simulink model "Scenario_MinimumExample_TwithoutTrafficLights_tol_fixed"  (R2021a)
settings: Solver=VariableStepAuto  StartTime=0.0  StopTime=50  RelTol=1e-3
model workspace (MAT data in the model file):
  Kz_dif : Simulink.Parameter (value not decoded)
  Kz_il : Simulink.Parameter (value not decoded)
  Kz_ir : Simulink.Parameter (value not decoded)
  Kz_is : Simulink.Parameter (value not decoded)
  Kz_long : Simulink.Parameter (value not decoded)
  Kz_pre : Simulink.Parameter (value not decoded)
  L_dif : Simulink.Parameter (value not decoded)
  L_il : Simulink.Parameter (value not decoded)
  L_ir : Simulink.Parameter (value not decoded)
  L_is : Simulink.Parameter (value not decoded)
  L_long : Simulink.Parameter (value not decoded)
  L_pre : Simulink.Parameter (value not decoded)
  Lc : Simulink.Parameter (value not decoded)
  Rk : Simulink.Parameter (value not decoded)
  Tz_dif : Simulink.Parameter (value not decoded)
  Tz_il : Simulink.Parameter (value not decoded)
  Tz_ir : Simulink.Parameter (value not decoded)
  Tz_is : Simulink.Parameter (value not decoded)
  Tz_long : Simulink.Parameter (value not decoded)
  Tz_pre : Simulink.Parameter (value not decoded)
  ds : Simulink.Parameter (value not decoded)
  dt : Simulink.Parameter (value not decoded)
  v : Simulink.Parameter (value not decoded)
symbols that are objects in the model workspace (value not decoded): Kz_dif, Kz_il, Kz_ir, Kz_is, Kz_long, Kz_pre, Rk, Tz_dif, Tz_il, Tz_ir, Tz_is, Tz_long, Tz_pre
libraries: StreetLanesLibrary x72, EdgesLibrary x64, MeasuringLibrary x34, SourcesAndSinksLibrary x11
(part 2 of 3)

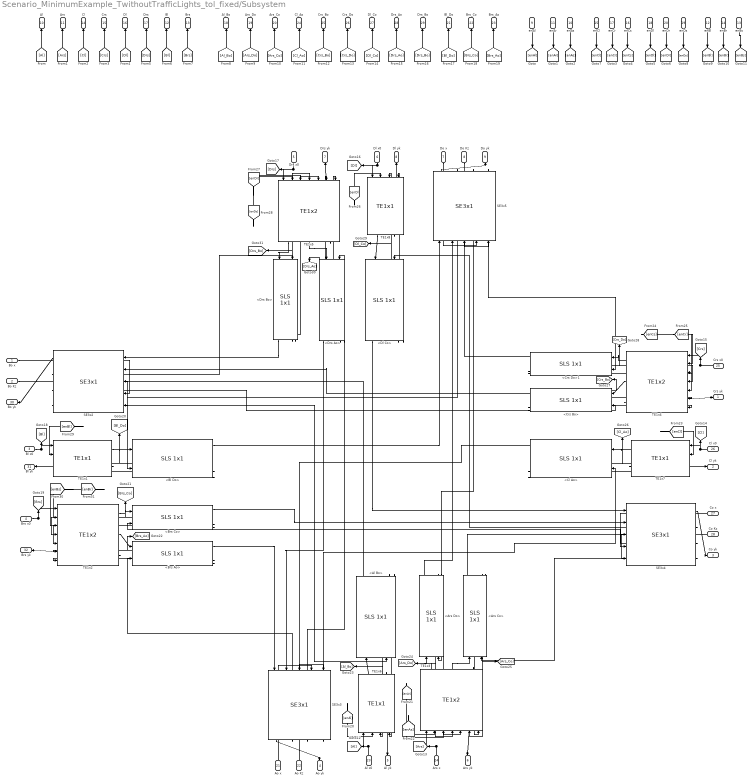
== system Scenario_MinimumExample_TwithoutTrafficLights_tol_fixed/Subsystem ==
  Bo x : Inport
  Bo Kz : Inport  Port=2
  Bl x0 : Inport  Port=3
  Brs x0 : Inport  Port=4
  Drs x0 : Inport  Port=5
  Dl x0 : Inport  Port=6
  Do x : Inport  Port=7
  Do Kz : Inport  Port=8
  enAl : Inport  Port=9
  enAs : Inport  Port=10
  enAr : Inport  Port=11
  enBl : Inport  Port=12
  enBs : Inport  Port=13
  enBr : Inport  Port=14
  enCl : Inport  Port=15
  enCs : Inport  Port=16
  enCr : Inport  Port=17
  enDl : Inport  Port=18
  enDs : Inport  Port=19
  enDr : Inport  Port=20
  Ao x : Inport  Port=21
  Ao Kz : Inport  Port=22
  Al x0 : Inport  Port=23
  Ars x : Inport  Port=24
  Crs x0 : Inport  Port=25
  Cl x0 : Inport  Port=26
  Co x : Inport  Port=27
  Co Kz : Inport  Port=28
  <Al Bo> : StreetLanesLibrary/SLS 1x1  Kz=Kz_left  Tz=Tz_left
  <Ars Co> : StreetLanesLibrary/SLS 1x1  Kz=Kz_right  Tz=Tz_right
  <Ars Do> : StreetLanesLibrary/SLS 1x1  Kz=Kz_straight  Tz=Tz_straight
  <Bl Do> : StreetLanesLibrary/SLS 1x1  Kz=Kz_left  Tz=Tz_left
  <Brs Ao> : StreetLanesLibrary/SLS 1x1  Kz=Kz_right  Tz=Tz_right
  <Brs Co> : StreetLanesLibrary/SLS 1x1  Kz=Kz_straight  Tz=Tz_straight
  <Cl Ao> : StreetLanesLibrary/SLS 1x1  Kz=Kz_left  Tz=Tz_left
  <Crs Bo> : StreetLanesLibrary/SLS 1x1  Kz=Kz_straight  Tz=Tz_straight
  <Crs Do>1 : StreetLanesLibrary/SLS 1x1  Kz=Kz_right  Tz=Tz_right
  <Dl Co> : StreetLanesLibrary/SLS 1x1  Kz=Kz_left  Tz=Tz_left
  <Drs Ao> : StreetLanesLibrary/SLS 1x1  Kz=Kz_straight  Tz=Tz_straight
  <Drs Bo> : StreetLanesLibrary/SLS 1x1  Kz=Kz_right  Tz=Tz_right
  SE3x{2..5} (4 alike) : EdgesLibrary/SE3x1  Rk1=Rk  Rk2=Rk  Rk3=Rk
  TE1x{1,6..8} (4 alike) : EdgesLibrary/TE1x1  Rk=Rk  slope=2000
  TE1x{2..5} (4 alike) : EdgesLibrary/TE1x2  Rk1=0.5*Rk  Rk2=0.5*Rk
  Crs yk : Outport
  Cl yk : Outport  Port=2
  Co yk : Outport  Port=3
  Ao yk : Outport  Port=4
  Al yk : Outport  Port=5
  Ars yk : Outport  Port=6
  Drs yk : Outport  Port=7
  Dl yk : Outport  Port=8
  Do yk : Outport  Port=9
  Al : Outport  Port=10
  Ars : Outport  Port=11
  Bl : Outport  Port=12
  Brs : Outport  Port=13
  Cl : Outport  Port=14
  Crs : Outport  Port=15
  Dl : Outport  Port=16
  Drs : Outport  Port=17
  Al_Bo : Outport  Port=18
  Ars_Do : Outport  Port=19
  Ars_Co : Outport  Port=20
  Bl_Do : Outport  Port=21
  Brs_Co : Outport  Port=22
  Brs_Ao : Outport  Port=23
  Cl_Ao : Outport  Port=24
  Crs_Bo : Outport  Port=25
  Crs_Do : Outport  Port=26
  Dl_Co : Outport  Port=27
  Drs_Ao : Outport  Port=28
  Drs_Bo : Outport  Port=29
  Bo yk : Outport  Port=30
  Bl yk : Outport  Port=31
  Brs yk : Outport  Port=32
  wires:
  SE3x2/1 -> Bo yk/1
  Bo Kz/1 -> SE3x2/5
  Bo x/1 -> SE3x2/4
  Bl x0/1 -> [Bl], TE1x1/1
  TE1x1/2 -> Bl yk/1
  Brs x0/1 -> [Brs], TE1x2/1
  TE1x2/3 -> Brs yk/1
  Ao x/1 -> SE3x3/4
  Ao Kz/1 -> SE3x3/5
  SE3x3/1 -> Ao yk/1
  Ars x/1 -> [Ars], TE1x3/1
  TE1x3/3 -> Ars yk/1
  Co Kz/1 -> SE3x4/5
  Co x/1 -> SE3x4/4
  SE3x4/1 -> Co yk/1
  TE1x4/3 -> Crs yk/1
  Crs x0/1 -> [Crs], TE1x4/1
  Do x/1 -> SE3x5/4
  Do Kz/1 -> SE3x5/5
  SE3x5/1 -> Do yk/1
  TE1x5/3 -> Drs yk/1
  Drs x0/1 -> [Drs], TE1x5/1
  TE1x4/2 -> <Crs Bo>/1
  <Crs Bo>/8 -> TE1x4/7
  <Crs Bo>/7 -> [Crs_Bo], TE1x4/6
  TE1x3/1 -> <Ars Do>/1
  <Ars Do>/8 -> TE1x3/5
  <Ars Do>/7 -> [Ars_Do], TE1x3/4
  TE1x2/1 -> <Brs Co>/1
  <Brs Co>/8 -> TE1x2/5
  <Brs Co>/7 -> [Brs_Co], TE1x2/4
  TE1x2/2 -> <Brs Ao>/1
  <Brs Ao>/8 -> TE1x2/7
  <Brs Ao>/7 -> TE1x2/6, [Brs_Ao]
  TE1x4/1 -> <Crs Do>1/1
  <Crs Do>1/8 -> TE1x4/5
  <Crs Do>1/7 -> [Crs_Do], TE1x4/4
  TE1x5/1 -> <Drs Bo>/1
  <Drs Bo>/8 -> TE1x5/5
  TE1x5/2 -> <Drs Ao>/1
  <Drs Ao>/8 -> TE1x5/7
  <Drs Ao>/7 -> [Drs_Ao], TE1x5/6
  TE1x3/2 -> <Ars Co>/1
  <Ars Co>/8 -> TE1x3/7
  TE1x1/1 -> <Bl Do>/1
  <Bl Do>/8 -> TE1x1/4
  <Bl Do>/7 -> [Bl_Do], TE1x1/3
  <Cl Ao>/7 -> TE1x7/3, [Cl_Ao]
  <Cl Ao>/8 -> TE1x7/4
  TE1x7/1 -> <Cl Ao>/1
  TE1x8/1 -> <Dl Co>/1
  <Dl Co>/8 -> TE1x8/4
  <Dl Co>/7 -> [Dl_Co], TE1x8/3
  TE1x6/1 -> <Al Bo>/1
  <Al Bo>/8 -> TE1x6/4
  <Al Bo>/7 -> TE1x6/3, [Al_Bo]
  <Drs Bo>/2 -> SE3x2/1
  SE3x2/2 -> <Drs Bo>/2
  <Crs Bo>/2 -> SE3x2/2
  SE3x2/3 -> <Crs Bo>/2
  <Al Bo>/2 -> SE3x2/3
  SE3x2/4 -> <Al Bo>/2
  <Crs Do>1/2 -> SE3x5/3
  SE3x5/4 -> <Crs Do>1/2
  SE3x5/3 -> <Ars Do>/2
  <Ars Do>/2 -> SE3x5/2
  <Bl Do>/2 -> SE3x5/1
  SE3x5/2 -> <Bl Do>/2
  SE3x4/4 -> <Ars Co>/2
  <Ars Co>/2 -> SE3x4/3
  SE3x4/3 -> <Brs Co>/2
  <Brs Co>/2 -> SE3x4/2
  SE3x4/2 -> <Dl Co>/2
  <Dl Co>/2 -> SE3x4/1
  SE3x3/2 -> <Brs Ao>/2
  <Brs Ao>/2 -> SE3x3/1
  SE3x3/3 -> <Drs Ao>/2
  <Drs Ao>/2 -> SE3x3/2
  SE3x3/4 -> <Cl Ao>/2
  <Cl Ao>/2 -> SE3x3/3
  <Ars Co>/7 -> TE1x3/6, [Ars_Co]
  Al x0/1 -> [Al], TE1x6/1
  TE1x6/2 -> Al yk/1
  Cl x0/1 -> [Cl], TE1x7/1
  TE1x7/2 -> Cl yk/1
  Dl x0/1 -> [Dl], TE1x8/1
  TE1x8/2 -> Dl yk/1
  [enAl] -> TE1x6/2
  [enAr] -> TE1x3/3
  [enAs] -> TE1x3/2
  [enCl] -> TE1x7/2
  [enCs] -> TE1x4/3
  [enCr] -> TE1x4/2
  [enDl] -> TE1x8/2
  [enBl] -> TE1x1/2
  [enBs] -> TE1x2/2
  [enBr] -> TE1x2/3
  [enDr] -> TE1x5/2
  [enDs] -> TE1x5/3
  <Drs Bo>/7 -> TE1x5/4, [Drs_Bo]
  [Al] -> Al/1
  [Ars] -> Ars/1
  [Cl] -> Cl/1
  [Crs] -> Crs/1
  [Dl] -> Dl/1
  [Drs] -> Drs/1
  [Bl] -> Bl/1
  [Brs] -> Brs/1
  [Al_Bo] -> Al_Bo/1
  [Ars_Do] -> Ars_Do/1
  [Ars_Co] -> Ars_Co/1
  [Cl_Ao] -> Cl_Ao/1
  [Crs_Bo] -> Crs_Bo/1
  [Crs_Do] -> Crs_Do/1
  [Dl_Co] -> Dl_Co/1
  [Drs_Ao] -> Drs_Ao/1
  [Drs_Bo] -> Drs_Bo/1
  [Bl_Do] -> Bl_Do/1
  [Brs_Co] -> Brs_Co/1
  [Brs_Ao] -> Brs_Ao/1
  enAl/1 -> [enAl]
  enAr/1 -> [enAr]
  enAs/1 -> [enAs]
  enCl/1 -> [enCl]
  enCr/1 -> [enCr]
  enCs/1 -> [enCs]
  enDl/1 -> [enDl]
  enDr/1 -> [enDr]
  enDs/1 -> [enDs]
  enBl/1 -> [enBl]
  enBr/1 -> [enBr]
  enBs/1 -> [enBs]

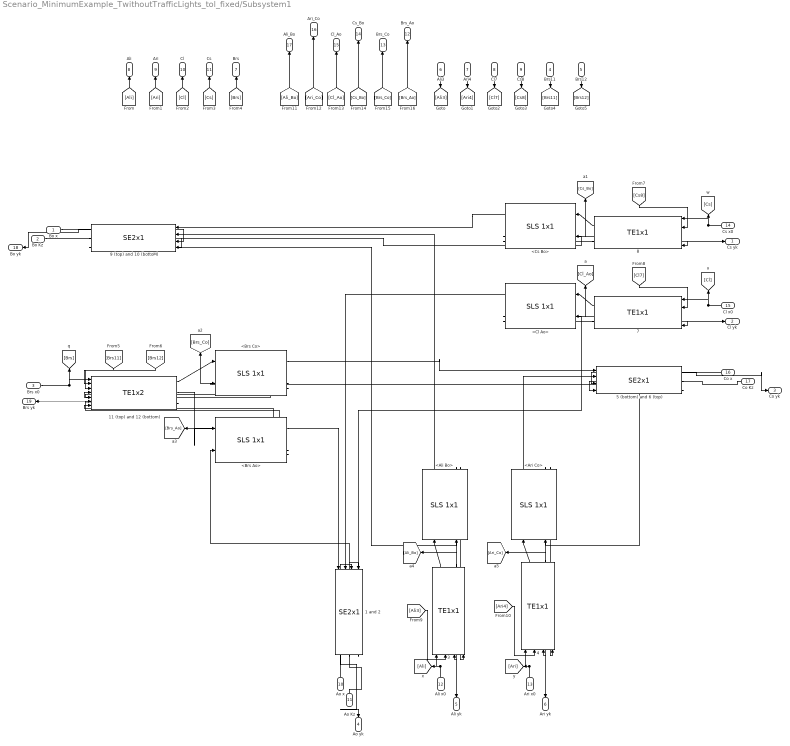
== system Scenario_MinimumExample_TwithoutTrafficLights_tol_fixed/Subsystem1 ==
  Bo x : Inport
  Bo Kz : Inport  Port=2
  Brs x0 : Inport  Port=3
  Brs11 : Inport  Port=4
  Brs12 : Inport  Port=5
  Ali3 : Inport  Port=6
  Ari4 : Inport  Port=7
  Cl7 : Inport  Port=8
  Cs8 : Inport  Port=9
  Ao x : Inport  Port=10
  Ao Kz : Inport  Port=11
  Ali x0 : Inport  Port=12
  Ari x0 : Inport  Port=13
  Cs x0 : Inport  Port=14
  Cl x0 : Inport  Port=15
  Co x : Inport  Port=16
  Co Kz : Inport  Port=17
  1 and 2 : EdgesLibrary/SE2x1  Rk1=Rk  Rk2=Rk
  11 (top) and 12 (bottom) : EdgesLibrary/TE1x2  Rk1=0.5*Rk  Rk2=0.5*Rk
  {3..4,7..8} (4 alike) : EdgesLibrary/TE1x1  Rk=Rk  slope=2000
  5 (bottom) and 6 (top) : EdgesLibrary/SE2x1  Rk1=Rk  Rk2=Rk
  9 (top) and 10 (bottoM) : EdgesLibrary/SE2x1  Rk1=Rk  Rk2=Rk
  <Ali Bo> : StreetLanesLibrary/SLS 1x1  Kz=Kz_left  Tz=Tz_left
  <Ari Co> : StreetLanesLibrary/SLS 1x1  Kz=Kz_right  Tz=Tz_right
  <Brs Ao> : StreetLanesLibrary/SLS 1x1  Kz=Kz_right  Tz=Tz_right
  <Brs Co> : StreetLanesLibrary/SLS 1x1  Kz=Kz_straight  Tz=Tz_straight
  <Cl Ao> : StreetLanesLibrary/SLS 1x1  Kz=Kz_left  Tz=Tz_left
  <Cs Bo> : StreetLanesLibrary/SLS 1x1  Kz=Kz_straight  Tz=Tz_straight
  Cs yk : Outport
  Cl yk : Outport  Port=2
  Co yk : Outport  Port=3
  Ao yk : Outport  Port=4
  Ali yk : Outport  Port=5
  Ari yk : Outport  Port=6
  Brs : Outport  Port=7
  Ali : Outport  Port=8
  Ari : Outport  Port=9
  Cl : Outport  Port=10
  Cs : Outport  Port=11
  Brs_Ao : Outport  Port=12
  Brs_Co : Outport  Port=13
  Cs_Bo : Outport  Port=14
  Cl_Ao : Outport  Port=15
  Ari_Co : Outport  Port=16
  Ali_Bo : Outport  Port=17
  Bo yk : Outport  Port=18
  Brs yk : Outport  Port=19
  wires:
  11 (top) and 12 (bottom)/2 -> <Brs Ao>/1
  11 (top) and 12 (bottom)/3 -> Brs yk/1
  3/2 -> Ali yk/1
  3/1 -> <Ali Bo>/1
  Ari x0/1 -> [Ari], 4/1
  <Cs Bo>/2 -> 9 (top) and 10 (bottoM)/1
  <Cs Bo>/8 -> 8/4
  <Cl Ao>/8 -> 7/4
  Co x/1 -> 5 (bottom) and 6 (top)/3
  5 (bottom) and 6 (top)/1 -> Co yk/1
  5 (bottom) and 6 (top)/3 -> <Ari Co>/2
  <Ari Co>/8 -> 4/4
  <Ali Bo>/8 -> 3/4
  Ao x/1 -> 1 and 2/3
  Brs x0/1 -> 11 (top) and 12 (bottom)/1, [Brs]
  <Brs Co>/2 -> 5 (bottom) and 6 (top)/1
  <Cl Ao>/7 -> [Cl_Ao], 7/3
  <Cl Ao>/2 -> 1 and 2/2
  9 (top) and 10 (bottoM)/2 -> <Cs Bo>/2
  <Ari Co>/2 -> 5 (bottom) and 6 (top)/2
  7/1 -> <Cl Ao>/1
  Cl x0/1 -> [Cl], 7/1
  4/1 -> <Ari Co>/1
  <Ari Co>/7 -> 4/3, [Ari_Co]
  <Brs Ao>/2 -> 1 and 2/1
  Ao Kz/1 -> 1 and 2/4
  <Brs Ao>/7 -> [Brs_Ao], 11 (top) and 12 (bottom)/6
  <Brs Ao>/8 -> 11 (top) and 12 (bottom)/7
  Co Kz/1 -> 5 (bottom) and 6 (top)/4
  8/2 -> Cs yk/1
  Bo Kz/1 -> 9 (top) and 10 (bottoM)/4
  1 and 2/3 -> <Cl Ao>/2
  <Brs Co>/8 -> 11 (top) and 12 (bottom)/5
  [Brs12] -> 11 (top) and 12 (bottom)/3
  9 (top) and 10 (bottoM)/3 -> <Ali Bo>/2
  <Ali Bo>/7 -> 3/3, [Ali_Bo]
  1 and 2/2 -> <Brs Ao>/2
  Ali x0/1 -> [Ali], 3/1
  <Brs Co>/7 -> 11 (top) and 12 (bottom)/4, [Brs_Co]
  1 and 2/1 -> Ao yk/1
  <Ali Bo>/2 -> 9 (top) and 10 (bottoM)/2
  [Ari4] -> 4/2
  5 (bottom) and 6 (top)/2 -> <Brs Co>/2
  8/1 -> <Cs Bo>/1
  4/2 -> Ari yk/1
  <Cs Bo>/7 -> 8/3, [Cs_Bo]
  Cs x0/1 -> [Cs], 8/1
  [Ali3] -> 3/2
  [Brs11] -> 11 (top) and 12 (bottom)/2
  11 (top) and 12 (bottom)/1 -> <Brs Co>/1
  Bo x/1 -> 9 (top) and 10 (bottoM)/3
  [Cl7] -> 7/2
  9 (top) and 10 (bottoM)/1 -> Bo yk/1
  7/2 -> Cl yk/1
  [Cs8] -> 8/2
  [Ali_Bo] -> Ali_Bo/1
  [Ari_Co] -> Ari_Co/1
  [Cl_Ao] -> Cl_Ao/1
  [Cs_Bo] -> Cs_Bo/1
  [Brs_Co] -> Brs_Co/1
  [Brs_Ao] -> Brs_Ao/1
  [Ali] -> Ali/1
  [Ari] -> Ari/1
  [Cl] -> Cl/1
  [Cs] -> Cs/1
  [Brs] -> Brs/1
  Ali3/1 -> [Ali3]
  Ari4/1 -> [Ari4]
  Cl7/1 -> [Cl7]
  Cs8/1 -> [Cs8]
  Brs11/1 -> [Brs11]
  Brs12/1 -> [Brs12]

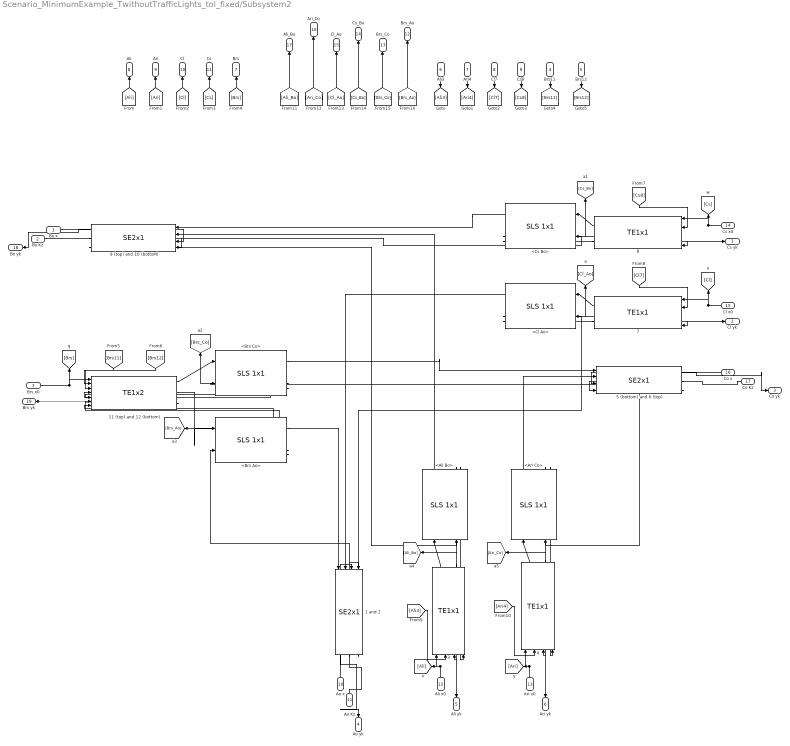
== system Scenario_MinimumExample_TwithoutTrafficLights_tol_fixed/Subsystem2 ==
  Bo x : Inport
  Bo Kz : Inport  Port=2
  Brs x0 : Inport  Port=3
  Brs11 : Inport  Port=4
  Brs12 : Inport  Port=5
  Ali3 : Inport  Port=6
  Ari4 : Inport  Port=7
  Cl7 : Inport  Port=8
  Cs8 : Inport  Port=9
  Ao x : Inport  Port=10
  Ao Kz : Inport  Port=11
  Ali x0 : Inport  Port=12
  Ari x0 : Inport  Port=13
  Cs x0 : Inport  Port=14
  Cl x0 : Inport  Port=15
  Co x : Inport  Port=16
  Co Kz : Inport  Port=17
  1 and 2 : EdgesLibrary/SE2x1  Rk1=Rk  Rk2=Rk
  11 (top) and 12 (bottom) : EdgesLibrary/TE1x2  Rk1=0.5*Rk  Rk2=0.5*Rk
  {3..4,7..8} (4 alike) : EdgesLibrary/TE1x1  Rk=Rk  slope=2000
  5 (bottom) and 6 (top) : EdgesLibrary/SE2x1  Rk1=Rk  Rk2=Rk
  9 (top) and 10 (bottoM) : EdgesLibrary/SE2x1  Rk1=Rk  Rk2=Rk
  <Ali Bo> : StreetLanesLibrary/SLS 1x1  Kz=Kz_left  Tz=Tz_left
  <Ari Co> : StreetLanesLibrary/SLS 1x1  Kz=Kz_right  Tz=Tz_right
  <Brs Ao> : StreetLanesLibrary/SLS 1x1  Kz=Kz_right  Tz=Tz_right
  <Brs Co> : StreetLanesLibrary/SLS 1x1  Kz=Kz_straight  Tz=Tz_straight
  <Cl Ao> : StreetLanesLibrary/SLS 1x1  Kz=Kz_left  Tz=Tz_left
  <Cs Bo> : StreetLanesLibrary/SLS 1x1  Kz=Kz_straight  Tz=Tz_straight
  Cs yk : Outport
  Cl yk : Outport  Port=2
  Co yk : Outport  Port=3
  Ao yk : Outport  Port=4
  Ali yk : Outport  Port=5
  Ari yk : Outport  Port=6
  Brs : Outport  Port=7
  Ali : Outport  Port=8
  Ari : Outport  Port=9
  Cl : Outport  Port=10
  Cs : Outport  Port=11
  Brs_Ao : Outport  Port=12
  Brs_Co : Outport  Port=13
  Cs_Bo : Outport  Port=14
  Cl_Ao : Outport  Port=15
  Ari_Co : Outport  Port=16
  Ali_Bo : Outport  Port=17
  Bo yk : Outport  Port=18
  Brs yk : Outport  Port=19
  wires:
  11 (top) and 12 (bottom)/2 -> <Brs Ao>/1
  11 (top) and 12 (bottom)/3 -> Brs yk/1
  3/2 -> Ali yk/1
  3/1 -> <Ali Bo>/1
  Ari x0/1 -> [Ari], 4/1
  <Cs Bo>/2 -> 9 (top) and 10 (bottoM)/1
  <Cs Bo>/8 -> 8/4
  <Cl Ao>/8 -> 7/4
  Co x/1 -> 5 (bottom) and 6 (top)/3
  5 (bottom) and 6 (top)/1 -> Co yk/1
  5 (bottom) and 6 (top)/3 -> <Ari Co>/2
  <Ari Co>/8 -> 4/4
  <Ali Bo>/8 -> 3/4
  Ao x/1 -> 1 and 2/3
  Brs x0/1 -> 11 (top) and 12 (bottom)/1, [Brs]
  <Brs Co>/2 -> 5 (bottom) and 6 (top)/1
  <Cl Ao>/7 -> [Cl_Ao], 7/3
  <Cl Ao>/2 -> 1 and 2/2
  9 (top) and 10 (bottoM)/2 -> <Cs Bo>/2
  <Ari Co>/2 -> 5 (bottom) and 6 (top)/2
  7/1 -> <Cl Ao>/1
  Cl x0/1 -> [Cl], 7/1
  4/1 -> <Ari Co>/1
  <Ari Co>/7 -> 4/3, [Ari_Co]
  <Brs Ao>/2 -> 1 and 2/1
  Ao Kz/1 -> 1 and 2/4
  <Brs Ao>/7 -> [Brs_Ao], 11 (top) and 12 (bottom)/6
  <Brs Ao>/8 -> 11 (top) and 12 (bottom)/7
  Co Kz/1 -> 5 (bottom) and 6 (top)/4
  8/2 -> Cs yk/1
  Bo Kz/1 -> 9 (top) and 10 (bottoM)/4
  1 and 2/3 -> <Cl Ao>/2
  <Brs Co>/8 -> 11 (top) and 12 (bottom)/5
  [Brs12] -> 11 (top) and 12 (bottom)/3
  9 (top) and 10 (bottoM)/3 -> <Ali Bo>/2
  <Ali Bo>/7 -> 3/3, [Ali_Bo]
  1 and 2/2 -> <Brs Ao>/2
  Ali x0/1 -> [Ali], 3/1
  <Brs Co>/7 -> 11 (top) and 12 (bottom)/4, [Brs_Co]
  1 and 2/1 -> Ao yk/1
  <Ali Bo>/2 -> 9 (top) and 10 (bottoM)/2
  [Ari4] -> 4/2
  5 (bottom) and 6 (top)/2 -> <Brs Co>/2
  8/1 -> <Cs Bo>/1
  4/2 -> Ari yk/1
  <Cs Bo>/7 -> 8/3, [Cs_Bo]
  Cs x0/1 -> [Cs], 8/1
  [Ali3] -> 3/2
  [Brs11] -> 11 (top) and 12 (bottom)/2
  11 (top) and 12 (bottom)/1 -> <Brs Co>/1
  Bo x/1 -> 9 (top) and 10 (bottoM)/3
  [Cl7] -> 7/2
  9 (top) and 10 (bottoM)/1 -> Bo yk/1
  7/2 -> Cl yk/1
  [Cs8] -> 8/2
  [Ali_Bo] -> Ali_Bo/1
  [Ari_Co] -> Ari_Co/1
  [Cl_Ao] -> Cl_Ao/1
  [Cs_Bo] -> Cs_Bo/1
  [Brs_Co] -> Brs_Co/1
  [Brs_Ao] -> Brs_Ao/1
  [Ali] -> Ali/1
  [Ari] -> Ari/1
  [Cl] -> Cl/1
  [Cs] -> Cs/1
  [Brs] -> Brs/1
  Ali3/1 -> [Ali3]
  Ari4/1 -> [Ari4]
  Cl7/1 -> [Cl7]
  Cs8/1 -> [Cs8]
  Brs11/1 -> [Brs11]
  Brs12/1 -> [Brs12]

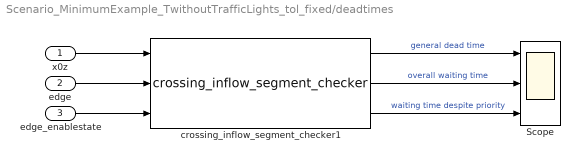
== system Scenario_MinimumExample_TwithoutTrafficLights_tol_fixed/deadtimes ==
  x0z : Inport
  edge : Inport  Port=2
  edge_enablestate : Inport  Port=3
  Scope : Scope  NumInputPorts=3
  crossing_inflow_segment_checker1 : MeasuringLibrary/crossing_inflow_segment_checker  SystemSampleTime=-1  VariantActivationTime=update diagram  Latency=0  AutoFrameSizeCalculation=off
  wires:
  crossing_inflow_segment_checker1/3 -> Scope/3  "waiting time despite priority"
  x0z/1 -> crossing_inflow_segment_checker1/1
  edge/1 -> crossing_inflow_segment_checker1/2
  crossing_inflow_segment_checker1/2 -> Scope/2  "overall waiting time"
  edge_enablestate/1 -> crossing_inflow_segment_checker1/3
  crossing_inflow_segment_checker1/1 -> Scope/1  "general dead time"

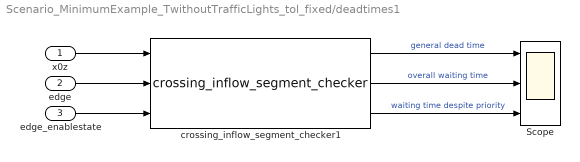
== system Scenario_MinimumExample_TwithoutTrafficLights_tol_fixed/deadtimes1 ==
  x0z : Inport
  edge : Inport  Port=2
  edge_enablestate : Inport  Port=3
  Scope : Scope  NumInputPorts=3
  crossing_inflow_segment_checker1 : MeasuringLibrary/crossing_inflow_segment_checker  SystemSampleTime=-1  VariantActivationTime=update diagram  Latency=0  AutoFrameSizeCalculation=off
  wires:
  crossing_inflow_segment_checker1/3 -> Scope/3  "waiting time despite priority"
  x0z/1 -> crossing_inflow_segment_checker1/1
  edge/1 -> crossing_inflow_segment_checker1/2
  crossing_inflow_segment_checker1/2 -> Scope/2  "overall waiting time"
  edge_enablestate/1 -> crossing_inflow_segment_checker1/3
  crossing_inflow_segment_checker1/1 -> Scope/1  "general dead time"

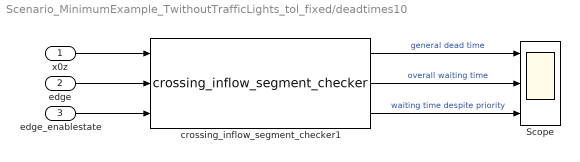
== system Scenario_MinimumExample_TwithoutTrafficLights_tol_fixed/deadtimes10 ==
  x0z : Inport
  edge : Inport  Port=2
  edge_enablestate : Inport  Port=3
  Scope : Scope  NumInputPorts=3
  crossing_inflow_segment_checker1 : MeasuringLibrary/crossing_inflow_segment_checker  SystemSampleTime=-1  VariantActivationTime=update diagram  Latency=0  AutoFrameSizeCalculation=off
  wires:
  crossing_inflow_segment_checker1/3 -> Scope/3  "waiting time despite priority"
  x0z/1 -> crossing_inflow_segment_checker1/1
  edge/1 -> crossing_inflow_segment_checker1/2
  crossing_inflow_segment_checker1/2 -> Scope/2  "overall waiting time"
  edge_enablestate/1 -> crossing_inflow_segment_checker1/3
  crossing_inflow_segment_checker1/1 -> Scope/1  "general dead time"

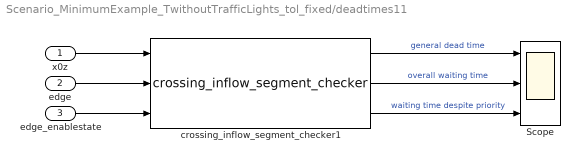
== system Scenario_MinimumExample_TwithoutTrafficLights_tol_fixed/deadtimes11 ==
  x0z : Inport
  edge : Inport  Port=2
  edge_enablestate : Inport  Port=3
  Scope : Scope  NumInputPorts=3
  crossing_inflow_segment_checker1 : MeasuringLibrary/crossing_inflow_segment_checker  SystemSampleTime=-1  VariantActivationTime=update diagram  Latency=0  AutoFrameSizeCalculation=off
  wires:
  crossing_inflow_segment_checker1/3 -> Scope/3  "waiting time despite priority"
  x0z/1 -> crossing_inflow_segment_checker1/1
  edge/1 -> crossing_inflow_segment_checker1/2
  crossing_inflow_segment_checker1/2 -> Scope/2  "overall waiting time"
  edge_enablestate/1 -> crossing_inflow_segment_checker1/3
  crossing_inflow_segment_checker1/1 -> Scope/1  "general dead time"

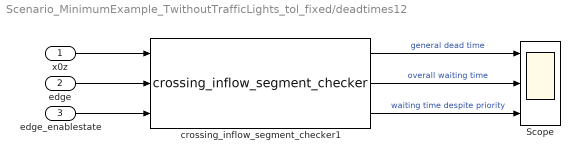
== system Scenario_MinimumExample_TwithoutTrafficLights_tol_fixed/deadtimes12 ==
  x0z : Inport
  edge : Inport  Port=2
  edge_enablestate : Inport  Port=3
  Scope : Scope  NumInputPorts=3
  crossing_inflow_segment_checker1 : MeasuringLibrary/crossing_inflow_segment_checker  SystemSampleTime=-1  VariantActivationTime=update diagram  Latency=0  AutoFrameSizeCalculation=off
  wires:
  crossing_inflow_segment_checker1/3 -> Scope/3  "waiting time despite priority"
  x0z/1 -> crossing_inflow_segment_checker1/1
  edge/1 -> crossing_inflow_segment_checker1/2
  crossing_inflow_segment_checker1/2 -> Scope/2  "overall waiting time"
  edge_enablestate/1 -> crossing_inflow_segment_checker1/3
  crossing_inflow_segment_checker1/1 -> Scope/1  "general dead time"

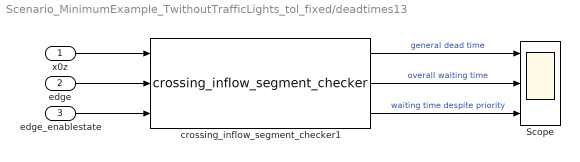
== system Scenario_MinimumExample_TwithoutTrafficLights_tol_fixed/deadtimes13 ==
  x0z : Inport
  edge : Inport  Port=2
  edge_enablestate : Inport  Port=3
  Scope : Scope  NumInputPorts=3
  crossing_inflow_segment_checker1 : MeasuringLibrary/crossing_inflow_segment_checker  SystemSampleTime=-1  VariantActivationTime=update diagram  Latency=0  AutoFrameSizeCalculation=off
  wires:
  crossing_inflow_segment_checker1/3 -> Scope/3  "waiting time despite priority"
  x0z/1 -> crossing_inflow_segment_checker1/1
  edge/1 -> crossing_inflow_segment_checker1/2
  crossing_inflow_segment_checker1/2 -> Scope/2  "overall waiting time"
  edge_enablestate/1 -> crossing_inflow_segment_checker1/3
  crossing_inflow_segment_checker1/1 -> Scope/1  "general dead time"

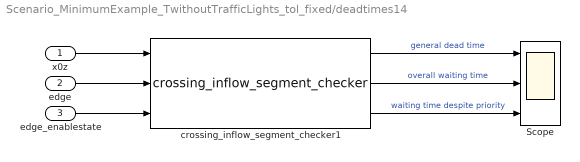
== system Scenario_MinimumExample_TwithoutTrafficLights_tol_fixed/deadtimes14 ==
  x0z : Inport
  edge : Inport  Port=2
  edge_enablestate : Inport  Port=3
  Scope : Scope  NumInputPorts=3
  crossing_inflow_segment_checker1 : MeasuringLibrary/crossing_inflow_segment_checker  SystemSampleTime=-1  VariantActivationTime=update diagram  Latency=0  AutoFrameSizeCalculation=off
  wires:
  crossing_inflow_segment_checker1/3 -> Scope/3  "waiting time despite priority"
  x0z/1 -> crossing_inflow_segment_checker1/1
  edge/1 -> crossing_inflow_segment_checker1/2
  crossing_inflow_segment_checker1/2 -> Scope/2  "overall waiting time"
  edge_enablestate/1 -> crossing_inflow_segment_checker1/3
  crossing_inflow_segment_checker1/1 -> Scope/1  "general dead time"

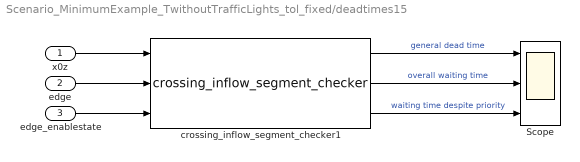
== system Scenario_MinimumExample_TwithoutTrafficLights_tol_fixed/deadtimes15 ==
  x0z : Inport
  edge : Inport  Port=2
  edge_enablestate : Inport  Port=3
  Scope : Scope  NumInputPorts=3
  crossing_inflow_segment_checker1 : MeasuringLibrary/crossing_inflow_segment_checker  SystemSampleTime=-1  VariantActivationTime=update diagram  Latency=0  AutoFrameSizeCalculation=off
  wires:
  crossing_inflow_segment_checker1/3 -> Scope/3  "waiting time despite priority"
  x0z/1 -> crossing_inflow_segment_checker1/1
  edge/1 -> crossing_inflow_segment_checker1/2
  crossing_inflow_segment_checker1/2 -> Scope/2  "overall waiting time"
  edge_enablestate/1 -> crossing_inflow_segment_checker1/3
  crossing_inflow_segment_checker1/1 -> Scope/1  "general dead time"

== system Scenario_MinimumExample_TwithoutTrafficLights_tol_fixed/deadtimes16 ==
  x0z : Inport
  edge : Inport  Port=2
  edge_enablestate : Inport  Port=3
  Scope : Scope  NumInputPorts=3
  crossing_inflow_segment_checker1 : MeasuringLibrary/crossing_inflow_segment_checker  SystemSampleTime=-1  VariantActivationTime=update diagram  Latency=0  AutoFrameSizeCalculation=off
  wires:
  crossing_inflow_segment_checker1/3 -> Scope/3  "waiting time despite priority"
  x0z/1 -> crossing_inflow_segment_checker1/1
  edge/1 -> crossing_inflow_segment_checker1/2
  crossing_inflow_segment_checker1/2 -> Scope/2  "overall waiting time"
  edge_enablestate/1 -> crossing_inflow_segment_checker1/3
  crossing_inflow_segment_checker1/1 -> Scope/1  "general dead time"

== system Scenario_MinimumExample_TwithoutTrafficLights_tol_fixed/deadtimes17 ==
  x0z : Inport
  edge : Inport  Port=2
  edge_enablestate : Inport  Port=3
  Scope : Scope  NumInputPorts=3
  crossing_inflow_segment_checker1 : MeasuringLibrary/crossing_inflow_segment_checker  SystemSampleTime=-1  VariantActivationTime=update diagram  Latency=0  AutoFrameSizeCalculation=off
  wires:
  crossing_inflow_segment_checker1/3 -> Scope/3  "waiting time despite priority"
  x0z/1 -> crossing_inflow_segment_checker1/1
  edge/1 -> crossing_inflow_segment_checker1/2
  crossing_inflow_segment_checker1/2 -> Scope/2  "overall waiting time"
  edge_enablestate/1 -> crossing_inflow_segment_checker1/3
  crossing_inflow_segment_checker1/1 -> Scope/1  "general dead time"

== system Scenario_MinimumExample_TwithoutTrafficLights_tol_fixed/deadtimes2 ==
  x0z : Inport
  edge : Inport  Port=2
  edge_enablestate : Inport  Port=3
  Scope : Scope  NumInputPorts=3
  crossing_inflow_segment_checker1 : MeasuringLibrary/crossing_inflow_segment_checker  SystemSampleTime=-1  VariantActivationTime=update diagram  Latency=0  AutoFrameSizeCalculation=off
  wires:
  crossing_inflow_segment_checker1/3 -> Scope/3  "waiting time despite priority"
  x0z/1 -> crossing_inflow_segment_checker1/1
  edge/1 -> crossing_inflow_segment_checker1/2
  crossing_inflow_segment_checker1/2 -> Scope/2  "overall waiting time"
  edge_enablestate/1 -> crossing_inflow_segment_checker1/3
  crossing_inflow_segment_checker1/1 -> Scope/1  "general dead time"

== system Scenario_MinimumExample_TwithoutTrafficLights_tol_fixed/deadtimes3 ==
  x0z : Inport
  edge : Inport  Port=2
  edge_enablestate : Inport  Port=3
  Scope : Scope  NumInputPorts=3
  crossing_inflow_segment_checker1 : MeasuringLibrary/crossing_inflow_segment_checker  SystemSampleTime=-1  VariantActivationTime=update diagram  Latency=0  AutoFrameSizeCalculation=off
  wires:
  crossing_inflow_segment_checker1/3 -> Scope/3  "waiting time despite priority"
  x0z/1 -> crossing_inflow_segment_checker1/1
  edge/1 -> crossing_inflow_segment_checker1/2
  crossing_inflow_segment_checker1/2 -> Scope/2  "overall waiting time"
  edge_enablestate/1 -> crossing_inflow_segment_checker1/3
  crossing_inflow_segment_checker1/1 -> Scope/1  "general dead time"

== system Scenario_MinimumExample_TwithoutTrafficLights_tol_fixed/deadtimes4 ==
  x0z : Inport
  edge : Inport  Port=2
  edge_enablestate : Inport  Port=3
  Scope : Scope  NumInputPorts=3
  crossing_inflow_segment_checker1 : MeasuringLibrary/crossing_inflow_segment_checker  SystemSampleTime=-1  VariantActivationTime=update diagram  Latency=0  AutoFrameSizeCalculation=off
  wires:
  crossing_inflow_segment_checker1/3 -> Scope/3  "waiting time despite priority"
  x0z/1 -> crossing_inflow_segment_checker1/1
  edge/1 -> crossing_inflow_segment_checker1/2
  crossing_inflow_segment_checker1/2 -> Scope/2  "overall waiting time"
  edge_enablestate/1 -> crossing_inflow_segment_checker1/3
  crossing_inflow_segment_checker1/1 -> Scope/1  "general dead time"

== system Scenario_MinimumExample_TwithoutTrafficLights_tol_fixed/deadtimes5 ==
  x0z : Inport
  edge : Inport  Port=2
  edge_enablestate : Inport  Port=3
  Scope : Scope  NumInputPorts=3
  crossing_inflow_segment_checker1 : MeasuringLibrary/crossing_inflow_segment_checker  SystemSampleTime=-1  VariantActivationTime=update diagram  Latency=0  AutoFrameSizeCalculation=off
  wires:
  crossing_inflow_segment_checker1/3 -> Scope/3  "waiting time despite priority"
  x0z/1 -> crossing_inflow_segment_checker1/1
  edge/1 -> crossing_inflow_segment_checker1/2
  crossing_inflow_segment_checker1/2 -> Scope/2  "overall waiting time"
  edge_enablestate/1 -> crossing_inflow_segment_checker1/3
  crossing_inflow_segment_checker1/1 -> Scope/1  "general dead time"

== system Scenario_MinimumExample_TwithoutTrafficLights_tol_fixed/deadtimes6 ==
  x0z : Inport
  edge : Inport  Port=2
  edge_enablestate : Inport  Port=3
  Scope : Scope  NumInputPorts=3
  crossing_inflow_segment_checker1 : MeasuringLibrary/crossing_inflow_segment_checker  SystemSampleTime=-1  VariantActivationTime=update diagram  Latency=0  AutoFrameSizeCalculation=off
  wires:
  crossing_inflow_segment_checker1/3 -> Scope/3  "waiting time despite priority"
  x0z/1 -> crossing_inflow_segment_checker1/1
  edge/1 -> crossing_inflow_segment_checker1/2
  crossing_inflow_segment_checker1/2 -> Scope/2  "overall waiting time"
  edge_enablestate/1 -> crossing_inflow_segment_checker1/3
  crossing_inflow_segment_checker1/1 -> Scope/1  "general dead time"

== system Scenario_MinimumExample_TwithoutTrafficLights_tol_fixed/deadtimes7 ==
  x0z : Inport
  edge : Inport  Port=2
  edge_enablestate : Inport  Port=3
  Scope : Scope  NumInputPorts=3
  crossing_inflow_segment_checker1 : MeasuringLibrary/crossing_inflow_segment_checker  SystemSampleTime=-1  VariantActivationTime=update diagram  Latency=0  AutoFrameSizeCalculation=off
  wires:
  crossing_inflow_segment_checker1/3 -> Scope/3  "waiting time despite priority"
  x0z/1 -> crossing_inflow_segment_checker1/1
  edge/1 -> crossing_inflow_segment_checker1/2
  crossing_inflow_segment_checker1/2 -> Scope/2  "overall waiting time"
  edge_enablestate/1 -> crossing_inflow_segment_checker1/3
  crossing_inflow_segment_checker1/1 -> Scope/1  "general dead time"

== system Scenario_MinimumExample_TwithoutTrafficLights_tol_fixed/deadtimes8 ==
  x0z : Inport
  edge : Inport  Port=2
  edge_enablestate : Inport  Port=3
  Scope : Scope  NumInputPorts=3
  crossing_inflow_segment_checker1 : MeasuringLibrary/crossing_inflow_segment_checker  SystemSampleTime=-1  VariantActivationTime=update diagram  Latency=0  AutoFrameSizeCalculation=off
  wires:
  crossing_inflow_segment_checker1/3 -> Scope/3  "waiting time despite priority"
  x0z/1 -> crossing_inflow_segment_checker1/1
  edge/1 -> crossing_inflow_segment_checker1/2
  crossing_inflow_segment_checker1/2 -> Scope/2  "overall waiting time"
  edge_enablestate/1 -> crossing_inflow_segment_checker1/3
  crossing_inflow_segment_checker1/1 -> Scope/1  "general dead time"

== system Scenario_MinimumExample_TwithoutTrafficLights_tol_fixed/deadtimes9 ==
  x0z : Inport
  edge : Inport  Port=2
  edge_enablestate : Inport  Port=3
  Scope : Scope  NumInputPorts=3
  crossing_inflow_segment_checker1 : MeasuringLibrary/crossing_inflow_segment_checker  SystemSampleTime=-1  VariantActivationTime=update diagram  Latency=0  AutoFrameSizeCalculation=off
  wires:
  crossing_inflow_segment_checker1/3 -> Scope/3  "waiting time despite priority"
  x0z/1 -> crossing_inflow_segment_checker1/1
  edge/1 -> crossing_inflow_segment_checker1/2
  crossing_inflow_segment_checker1/2 -> Scope/2  "overall waiting time"
  edge_enablestate/1 -> crossing_inflow_segment_checker1/3
  crossing_inflow_segment_checker1/1 -> Scope/1  "general dead time"

== system Scenario_MinimumExample_TwithoutTrafficLights_tol_fixed/rel xz ==
  xz : Inport
  kz : Inport  Port=2
  Scope : Scope
  rel xz1 : MeasuringLibrary/rel xz  SystemSampleTime=-1  VariantActivationTime=update diagram  Latency=0  AutoFrameSizeCalculation=off
  wires:
  xz/1 -> rel xz1/1
  rel xz1/1 -> Scope/1  "relative xz"
  kz/1 -> rel xz1/2

== system Scenario_MinimumExample_TwithoutTrafficLights_tol_fixed/sinks ==
  edge : Inport
  Scope : Scope  NumInputPorts=2
  sink_edge_checker1 : MeasuringLibrary/sink_edge_checker  shortestPathTz=0
  wires:
  sink_edge_checker1/1 -> Scope/1  "maximum outflow time"
  edge/1 -> sink_edge_checker1/1
  sink_edge_checker1/2 -> Scope/2  "actual outflow time"

== system Scenario_MinimumExample_TwithoutTrafficLights_tol_fixed/sinks1 ==
  edge : Inport
  Scope : Scope  NumInputPorts=2
  sink_edge_checker1 : MeasuringLibrary/sink_edge_checker  shortestPathTz=shortestPathTz
  wires:
  sink_edge_checker1/1 -> Scope/1  "maximum outflow time"
  edge/1 -> sink_edge_checker1/1
  sink_edge_checker1/2 -> Scope/2  "actual outflow time"

== system Scenario_MinimumExample_TwithoutTrafficLights_tol_fixed/sinks2 ==
  edge : Inport
  Scope : Scope  NumInputPorts=2
  sink_edge_checker1 : MeasuringLibrary/sink_edge_checker  shortestPathTz=shortestPathTz
  wires:
  sink_edge_checker1/1 -> Scope/1  "maximum outflow time"
  edge/1 -> sink_edge_checker1/1
  sink_edge_checker1/2 -> Scope/2  "actual outflow time"

== system Scenario_MinimumExample_TwithoutTrafficLights_tol_fixed/sinks3 ==
  edge : Inport
  Scope : Scope  NumInputPorts=2
  sink_edge_checker1 : MeasuringLibrary/sink_edge_checker  shortestPathTz=shortestPathTz
  wires:
  sink_edge_checker1/1 -> Scope/1  "maximum outflow time"
  edge/1 -> sink_edge_checker1/1
  sink_edge_checker1/2 -> Scope/2  "actual outflow time"

== system Scenario_MinimumExample_TwithoutTrafficLights_tol_fixed/sinks4 ==
  edge : Inport
  Scope : Scope  NumInputPorts=2
  sink_edge_checker1 : MeasuringLibrary/sink_edge_checker  shortestPathTz=shortestPathTz
  wires:
  sink_edge_checker1/1 -> Scope/1  "maximum outflow time"
  edge/1 -> sink_edge_checker1/1
  sink_edge_checker1/2 -> Scope/2  "actual outflow time"

== system Scenario_MinimumExample_TwithoutTrafficLights_tol_fixed/sinks5 ==
  edge : Inport
  Scope : Scope  NumInputPorts=2
  sink_edge_checker1 : MeasuringLibrary/sink_edge_checker  shortestPathTz=shortestPathTz
  wires:
  sink_edge_checker1/1 -> Scope/1  "maximum outflow time"
  edge/1 -> sink_edge_checker1/1
  sink_edge_checker1/2 -> Scope/2  "actual outflow time"

== system Scenario_MinimumExample_TwithoutTrafficLights_tol_fixed/sinks6 ==
  edge : Inport
  Scope : Scope  NumInputPorts=2
  sink_edge_checker1 : MeasuringLibrary/sink_edge_checker  shortestPathTz=shortestPathTz
  wires:
  sink_edge_checker1/1 -> Scope/1  "maximum outflow time"
  edge/1 -> sink_edge_checker1/1
  sink_edge_checker1/2 -> Scope/2  "actual outflow time"

== system Scenario_MinimumExample_TwithoutTrafficLights_tol_fixed/sources ==
  edge : Inport
  Scope : Scope  NumInputPorts=2
  source_edge_checker1 : MeasuringLibrary/source_edge_checker  SystemSampleTime=-1  VariantActivationTime=update diagram  Latency=0  AutoFrameSizeCalculation=off
  wires:
  source_edge_checker1/1 -> Scope/1  "maximum inflow time"
  source_edge_checker1/2 -> Scope/2  "actual inflow time"
  edge/1 -> source_edge_checker1/1

== system Scenario_MinimumExample_TwithoutTrafficLights_tol_fixed/sources1 ==
  edge : Inport
  Scope : Scope  NumInputPorts=2
  source_edge_checker1 : MeasuringLibrary/source_edge_checker  SystemSampleTime=-1  VariantActivationTime=update diagram  Latency=0  AutoFrameSizeCalculation=off
  wires:
  source_edge_checker1/1 -> Scope/1  "maximum inflow time"
  source_edge_checker1/2 -> Scope/2  "actual inflow time"
  edge/1 -> source_edge_checker1/1

== system Scenario_MinimumExample_TwithoutTrafficLights_tol_fixed/sources2 ==
  edge : Inport
  Scope : Scope  NumInputPorts=2
  source_edge_checker1 : MeasuringLibrary/source_edge_checker  SystemSampleTime=-1  VariantActivationTime=update diagram  Latency=0  AutoFrameSizeCalculation=off
  wires:
  source_edge_checker1/1 -> Scope/1  "maximum inflow time"
  source_edge_checker1/2 -> Scope/2  "actual inflow time"
  edge/1 -> source_edge_checker1/1

== system Scenario_MinimumExample_TwithoutTrafficLights_tol_fixed/sources3 ==
  edge : Inport
  Scope : Scope  NumInputPorts=2
  source_edge_checker1 : MeasuringLibrary/source_edge_checker  SystemSampleTime=-1  VariantActivationTime=update diagram  Latency=0  AutoFrameSizeCalculation=off
  wires:
  source_edge_checker1/1 -> Scope/1  "maximum inflow time"
  source_edge_checker1/2 -> Scope/2  "actual inflow time"
  edge/1 -> source_edge_checker1/1

== system Scenario_MinimumExample_TwithoutTrafficLights_tol_fixed/sources4 ==
  edge : Inport
  Scope : Scope  NumInputPorts=2
  source_edge_checker1 : MeasuringLibrary/source_edge_checker  SystemSampleTime=-1  VariantActivationTime=update diagram  Latency=0  AutoFrameSizeCalculation=off
  wires:
  source_edge_checker1/1 -> Scope/1  "maximum inflow time"
  source_edge_checker1/2 -> Scope/2  "actual inflow time"
  edge/1 -> source_edge_checker1/1

== system Scenario_MinimumExample_TwithoutTrafficLights_tol_fixed/sources5 ==
  edge : Inport
  Scope : Scope  NumInputPorts=2
  source_edge_checker1 : MeasuringLibrary/source_edge_checker  SystemSampleTime=-1  VariantActivationTime=update diagram  Latency=0  AutoFrameSizeCalculation=off
  wires:
  source_edge_checker1/1 -> Scope/1  "maximum inflow time"
  source_edge_checker1/2 -> Scope/2  "actual inflow time"
  edge/1 -> source_edge_checker1/1

== system Scenario_MinimumExample_TwithoutTrafficLights_tol_fixed/sources6 ==
  edge : Inport
  Scope : Scope  NumInputPorts=2
  source_edge_checker1 : MeasuringLibrary/source_edge_checker  SystemSampleTime=-1  VariantActivationTime=update diagram  Latency=0  AutoFrameSizeCalculation=off
  wires:
  source_edge_checker1/1 -> Scope/1  "maximum inflow time"
  source_edge_checker1/2 -> Scope/2  "actual inflow time"
  edge/1 -> source_edge_checker1/1

== system Scenario_MinimumExample_TwithoutTrafficLights_tol_fixed/sources7 ==
  edge : Inport
  Scope : Scope  NumInputPorts=2
  source_edge_checker1 : MeasuringLibrary/source_edge_checker  SystemSampleTime=-1  VariantActivationTime=update diagram  Latency=0  AutoFrameSizeCalculation=off
  wires:
  source_edge_checker1/1 -> Scope/1  "maximum inflow time"
  source_edge_checker1/2 -> Scope/2  "actual inflow time"
  edge/1 -> source_edge_checker1/1

== stateflow chart Scenario_MinimumExample_TwithoutTrafficLights_tol_fixed/Chart1 ==
  note: Notizen (mal auf Deutsch):
      | wenn an einer kante etwas anliegt und keine der stärkeren kanten etwas anliegen hat,
      | und die konfliktbereiche frei sind: schalte kante frei
      | <Ali 3> wird dominiert von <Cl 7> und <Cs 8> [Kreuzungen: <Brs Co> <Cl Ao> <Cs Bo>
      | <Ari 4> wird nicht dominiert [Kreuzungen: <Brs Co>
      | <Cl 7> wird dominiert von <Brs 11> und <Brs 12> [Kreuzungen: <Brs Co> <Brs Ao><Ali Bo>
      | <Cs 8> wird nicht dominiert [Kreuzungen: <Ali Bo>
      | <Brs 11> wird dominiert von <Ali 3> und <Ari 4> [Kreuzungen: <Brs Ao> <Ali Bo> <Ari Co>*<Cl Ao>
      | <Brs 12> wird nicht dominiert [Kreuzungen: <Cl Ao>
      |
      | Anmerkung: die einflüsse Brs11 und Brs12 behindern sich nicht. da beide kanten an
      | EIN UND DEMSELBEN SEGMENT liegen, und unsere 0.5:0.5 gewichtung schon suggeriert,
      | dass sich hier die autos "spalten", können sich die autos beim "Parallelen" fließen
      | in die segmente <Brs Co> und <Brs Ao> nicht wirklich in die quere kommen. Oder selbst wenn sie es
      | tun, können wir nichts dagegen unternehmen - wenn wir einem der pfade gegenüber dem anderen
      | priorität geben, wird bei dem anderen jeweils NIE etwas fließen. Damit müssen wir wohl leben :(
      |
      | a)
      | if [Ali > 0 && Cl == 0 && Cs == 0 && Brs_Co == 0 && Cl_Ao == 0 && Cs_Bo == 0]{enableAli3=1;}
      | else {enableAli3=0;}
      | b)
      | if [Ari > 0 && Brs_Co == 0]{enableAri4=1;}
      | else {enableAri4=0;}
      | c)
      | if [Cl > 0 && Brs == 0 && Brs_Co == 0 && Brs_Ao == 0 && Ali_Bo == 0]{enableCl7=1;}
      | else {enableCl7=0;}
      | d)
      | if [Cs > 0 && Ali_Bo == 0]{enableCs8=1;}
      | else {enableCs8=0;}
      | e)
      | if [Brs > 0 && Ali == 0 && Ari == 0 && Ali_Bo == 0 && Ari_Co == 0 && Cl_Ao]{enableBrs11=1;}
      | else {enableBrs11=0;}
      | f)
      | if [Brs > 0 && Cl_Ao == 0]{enableBrs12=1;}
      | else {enableBrs12=0;}
      |
      | Anmerkung: Da es im Falle [Ali > 0 && Brs > 0 && Cl > 0] einen deadlock gibt, müssen wir uns entscheiden, wer fahren darf.
      |
      | // Brs11 soll das fahrtrecht bekommen, um den fluss entlang der geraden aufrechtzuerhalten, wenn möglich
      | if [Ari == 0 && (Ali_Bo == 0 && Ari_Co == 0 && Cl_Ao == 0)]{enableBrs11=1;}
      | else
      |
      | // falls Brs12 nicht kann, versucht Ali zu fahren. Eigentlich müsste Cl die nächstbeste Wahl sein,
      | // allerdings kann Cl im falle eines Deadlocks ohnehin nicht fließen, da wegen unserer modellierung
      | // der 1x2 kanten (bzw. 1x2 segmente) gilt "Deadlock => [Brs > 0] => [Brs12 will aktiv sein]" - und da
      | // Brs12 vorrang vor Cl7 hat, ist Cl7 in diesem szenario grundsätzlich blockiert.
      | if [Cs == 0 && (Brs_Co == 0 && Cl_Ao == 0 && Cs_Bo == 0)]{enableAli3=1;}
      | else //guess noone can make it
  note: ?
  state InitiatePerStepCheck
  note: Brs-11-<Brs Co>-6-Co
      | (Links will geradeaus)
  note: Brs-12-<Brs Ao>-1-Ao
      | (Links will geradeaus)
  note: Ari-4-<Ari Co>-5-Co
      | (Unten will rechts abbiegen)
  note: Cl-7-<Cl Ao>-2-Ao
      | (Rechts will links abbiegen)
  note: Cs-8-<Cl Ao>-9-Bo
      | (Rechts will geradeaus)
  note: Ali-3-<Ali Bo>-10-Bo
      | (Unten will Links abbiegen)
  note: Deadlock-Detection
  note: Anstelle der ebene für deadlock resolution konnte man den "Links will geradeaus" bereich in der reihenfolge VOR "Unten will links abbiegen" setzen. "Links will geradeaus" muss dann um eine weitere kante mit höchster priorität ergänzt werden mit einem label
      | [ (Ali > 0 && Brs > 0 && Cl > 0 ) && (Ari == 0 && Ali_Bo == 0 && Ari_Co == 0]{enableBrs11=1;}
      |
      | "Unten will links abbiegen" wird dann ebenfalls um eine Kante mit höchster priorität ergänzt mit dem Label
      | [ (Ali > 0 && Brs > 0 && Cl > 0) && (Cs_Bo == 0 && Cl_Ao == 0) && ~(enableBrs11==1)
  note: Deadlock-Resolution
  InitiatePerStepCheck -> (junction 23) [order 1] : [Ali > 0 && Cl == 0 && Cs == 0 && Brs_Co <= tol && Cl_Ao <= tol && Cs_Bo <= tol]
      | {enableAli3=1; }
  (junction 23) -> (junction 29) [order 1] : [Ari > 0 && Brs_Co <= tol]{enableAri4=1;}
  (junction 29) -> (junction 36) [order 1] : [Cl > 0 && Brs == 0 && Brs_Co <= tol && Brs_Ao <= tol && Ali_Bo <= tol]{enableCl7=1; }
  (junction 39) -> (junction 40) [order 1] : [Brs > 0 && Ali == 0 && Ari == 0 && Ali_Bo <= tol && Ari_Co <= tol && Cl_Ao <= tol]{enableBrs11=1;}
  (junction 40) -> (junction 45) [order 1] : [Brs > 0 && Cl_Ao <= tol]{enableBrs12=1;}
  (junction 36) -> (junction 39) [order 1] : [Cs > 0 && Ali_Bo <= tol]{enableCs8=1;}
  (junction 39) -> (junction 40) [order 2] : {enableBrs11=0;}
  (junction 29) -> (junction 36) [order 2] : {enableCl7=0;}
  (junction 36) -> (junction 39) [order 2] : {enableCs8=0;}
  (junction 23) -> (junction 29) [order 2] : {enableAri4=0;}
  (junction 40) -> (junction 45) [order 2] : {enableBrs12=0;}
  InitiatePerStepCheck -> (junction 23) [order 2] : {enableAli3=0;}
  (junction 45) -> (junction 53)
  (junction 53) -> InitiatePerStepCheck [order 2]
  (default) -> InitiatePerStepCheck : {enableAli3 = 0; enableAri4 = 0;
      | enableCl7 = 0; enableCs8 = 0;
      | enableBrs11 = 0; enableBrs12 = 0;}
  (junction 53) -> (junction 64) [order 1] : [Ali > 0 && Brs > 0 && Cl > 0]
  (junction 64) -> (junction 71) [order 1] : [Ari == 0 && (Ali_Bo <= tol && Ari_Co <= tol && Cl_Ao <= tol)]{enableBrs11=1;}
  (junction 64) -> (junction 71) [order 2] : [Ari > 0 && Cs == 0 && (Brs_Co <= tol && Cl_Ao <= tol && Cs_Bo <= tol)]{enableAli3=1;}
  (junction 71) -> InitiatePerStepCheck
  data: Ali input; Ari input; Cl input; Cs input; Brs input; Ali_Bo input; Ari_Co input; Cl_Ao input; Cs_Bo input; Brs_Co input; Brs_Ao input; enableAli3 output; enableAri4 output; enableCl7 output; enableCs8 output; enableBrs11 output; enableBrs12 output; tol parameter

== stateflow chart Scenario_MinimumExample_TwithoutTrafficLights_tol_fixed/Chart2 ==
  note: Notizen (mal auf Deutsch):
      | wenn an einer kante etwas anliegt und keine der stärkeren kanten etwas anliegen hat,
      | und die konfliktbereiche frei sind: schalte kante frei
      | <Ali 3> wird dominiert von <Cl 7> und <Cs 8> [Kreuzungen: <Brs Co> <Cl Ao> <Cs Bo>
      | <Ari 4> wird nicht dominiert [Kreuzungen: <Brs Co>
      | <Cl 7> wird dominiert von <Brs 11> und <Brs 12> [Kreuzungen: <Brs Co> <Brs Ao><Ali Bo>
      | <Cs 8> wird nicht dominiert [Kreuzungen: <Ali Bo>
      | <Brs 11> wird dominiert von <Ali 3> und <Ari 4> [Kreuzungen: <Brs Ao> <Ali Bo> <Ari Co>*<Cl Ao>
      | <Brs 12> wird nicht dominiert [Kreuzungen: <Cl Ao>
      |
      | Anmerkung: die einflüsse Brs11 und Brs12 behindern sich nicht. da beide kanten an
      | EIN UND DEMSELBEN SEGMENT liegen, und unsere 0.5:0.5 gewichtung schon suggeriert,
      | dass sich hier die autos "spalten", können sich die autos beim "Parallelen" fließen
      | in die segmente <Brs Co> und <Brs Ao> nicht wirklich in die quere kommen. Oder selbst wenn sie es
      | tun, können wir nichts dagegen unternehmen - wenn wir einem der pfade gegenüber dem anderen
      | priorität geben, wird bei dem anderen jeweils NIE etwas fließen. Damit müssen wir wohl leben :(
      |
      | a)
      | if [Ali > 0 && Cl == 0 && Cs == 0 && Brs_Co == 0 && Cl_Ao == 0 && Cs_Bo == 0]{enableAli3=1;}
      | else {enableAli3=0;}
      | b)
      | if [Ari > 0 && Brs_Co == 0]{enableAri4=1;}
      | else {enableAri4=0;}
      | c)
      | if [Cl > 0 && Brs == 0 && Brs_Co == 0 && Brs_Ao == 0 && Ali_Bo == 0]{enableCl7=1;}
      | else {enableCl7=0;}
      | d)
      | if [Cs > 0 && Ali_Bo == 0]{enableCs8=1;}
      | else {enableCs8=0;}
      | e)
      | if [Brs > 0 && Ali == 0 && Ari == 0 && Ali_Bo == 0 && Ari_Co == 0 && Cl_Ao]{enableBrs11=1;}
      | else {enableBrs11=0;}
      | f)
      | if [Brs > 0 && Cl_Ao == 0]{enableBrs12=1;}
      | else {enableBrs12=0;}
      |
      | Anmerkung: Da es im Falle [Ali > 0 && Brs > 0 && Cl > 0] einen deadlock gibt, müssen wir uns entscheiden, wer fahren darf.
      |
      | // Brs11 soll das fahrtrecht bekommen, um den fluss entlang der geraden aufrechtzuerhalten, wenn möglich
      | if [Ari == 0 && (Ali_Bo == 0 && Ari_Co == 0 && Cl_Ao == 0)]{enableBrs11=1;}
      | else
      |
      | // falls Brs12 nicht kann, versucht Ali zu fahren. Eigentlich müsste Cl die nächstbeste Wahl sein,
      | // allerdings kann Cl im falle eines Deadlocks ohnehin nicht fließen, da wegen unserer modellierung
      | // der 1x2 kanten (bzw. 1x2 segmente) gilt "Deadlock => [Brs > 0] => [Brs12 will aktiv sein]" - und da
      | // Brs12 vorrang vor Cl7 hat, ist Cl7 in diesem szenario grundsätzlich blockiert.
      | if [Cs == 0 && (Brs_Co == 0 && Cl_Ao == 0 && Cs_Bo == 0)]{enableAli3=1;}
      | else //guess noone can make it
  note: ?
  state InitiatePerStepCheck
  note: Brs-11-<Brs Co>-6-Co
      | (Links will geradeaus)
  note: Brs-12-<Brs Ao>-1-Ao
      | (Links will geradeaus)
  note: Ari-4-<Ari Co>-5-Co
      | (Unten will rechts abbiegen)
  note: Cl-7-<Cl Ao>-2-Ao
      | (Rechts will links abbiegen)
  note: Cs-8-<Cl Ao>-9-Bo
      | (Rechts will geradeaus)
  note: Ali-3-<Ali Bo>-10-Bo
      | (Unten will Links abbiegen)
  note: Deadlock-Detection
  note: Anstelle der ebene für deadlock resolution konnte man den "Links will geradeaus" bereich in der reihenfolge VOR "Unten will links abbiegen" setzen. "Links will geradeaus" muss dann um eine weitere kante mit höchster priorität ergänzt werden mit einem label
      | [ (Ali > 0 && Brs > 0 && Cl > 0 ) && (Ari == 0 && Ali_Bo == 0 && Ari_Co == 0]{enableBrs11=1;}
      |
      | "Unten will links abbiegen" wird dann ebenfalls um eine Kante mit höchster priorität ergänzt mit dem Label
      | [ (Ali > 0 && Brs > 0 && Cl > 0) && (Cs_Bo == 0 && Cl_Ao == 0) && ~(enableBrs11==1)
  note: Deadlock-Resolution
  InitiatePerStepCheck -> (junction 23) [order 1] : [Ali > 0 && Cl == 0 && Cs == 0 && Brs_Co <= tol && Cl_Ao <= tol && Cs_Bo <= tol]
      | {enableAli3=1; }
  (junction 23) -> (junction 29) [order 1] : [Ari > 0 && Brs_Co <= tol]{enableAri4=1;}
  (junction 29) -> (junction 36) [order 1] : [Cl > 0 && Brs == 0 && Brs_Co <= tol && Brs_Ao <= tol && Ali_Bo <= tol]{enableCl7=1; }
  (junction 39) -> (junction 40) [order 1] : [Brs > 0 && Ali == 0 && Ari == 0 && Ali_Bo <= tol && Ari_Co <= tol && Cl_Ao <= tol]{enableBrs11=1;}
  (junction 40) -> (junction 45) [order 1] : [Brs > 0 && Cl_Ao <= tol]{enableBrs12=1;}
  (junction 36) -> (junction 39) [order 1] : [Cs > 0 && Ali_Bo <= tol]{enableCs8=1;}
  (junction 39) -> (junction 40) [order 2] : {enableBrs11=0;}
  (junction 29) -> (junction 36) [order 2] : {enableCl7=0;}
  (junction 36) -> (junction 39) [order 2] : {enableCs8=0;}
  (junction 23) -> (junction 29) [order 2] : {enableAri4=0;}
  (junction 40) -> (junction 45) [order 2] : {enableBrs12=0;}
  InitiatePerStepCheck -> (junction 23) [order 2] : {enableAli3=0;}
  (junction 45) -> (junction 53)
  (junction 53) -> InitiatePerStepCheck [order 2]
  (default) -> InitiatePerStepCheck : {enableAli3 = 0; enableAri4 = 0;
      | enableCl7 = 0; enableCs8 = 0;
      | enableBrs11 = 0; enableBrs12 = 0;}
  (junction 53) -> (junction 64) [order 1] : [Ali > 0 && Brs > 0 && Cl > 0]
  (junction 64) -> (junction 71) [order 1] : [Ari == 0 && (Ali_Bo <= tol && Ari_Co <= tol && Cl_Ao <= tol)]{enableBrs11=1;}
  (junction 64) -> (junction 71) [order 2] : [Ari > 0 && Cs == 0 && (Brs_Co <= tol && Cl_Ao <= tol && Cs_Bo <= tol)]{enableAli3=1;}
  (junction 71) -> InitiatePerStepCheck
  data: Ali input; Ari input; Cl input; Cs input; Brs input; Ali_Bo input; Ari_Co input; Cl_Ao input; Cs_Bo input; Brs_Co input; Brs_Ao input; enableAli3 output; enableAri4 output; enableCl7 output; enableCs8 output; enableBrs11 output; enableBrs12 output; tol parameter
